simulink subsystem "F550_Dynamic_CA"  (R2024a)
settings: Solver=VariableStepAuto  StartTime=0.0  StopTime=10.0  RelTol=1e-3
values from neighbouring files (symbols this model uses):
  Jxx = 0.0211    [F550_data.m]
  Jyy = 0.0219    [F550_data.m]
  Jzz = 0.0366    [F550_data.m]
  Mass = 2.06    [F550_data.m]
settings Model: Creator=UASG  LastModifiedBy=UASG

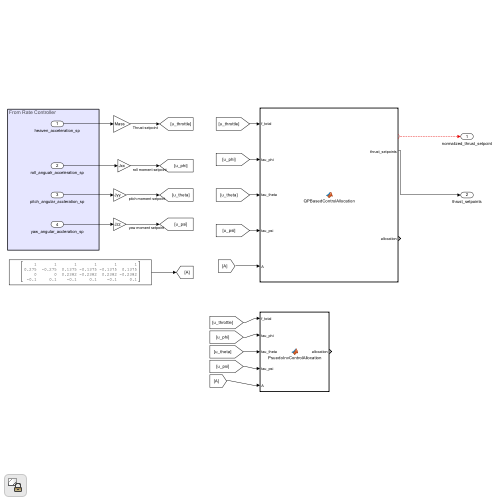
[thumbnail: Simulink's stored preview of the top-level diagram]
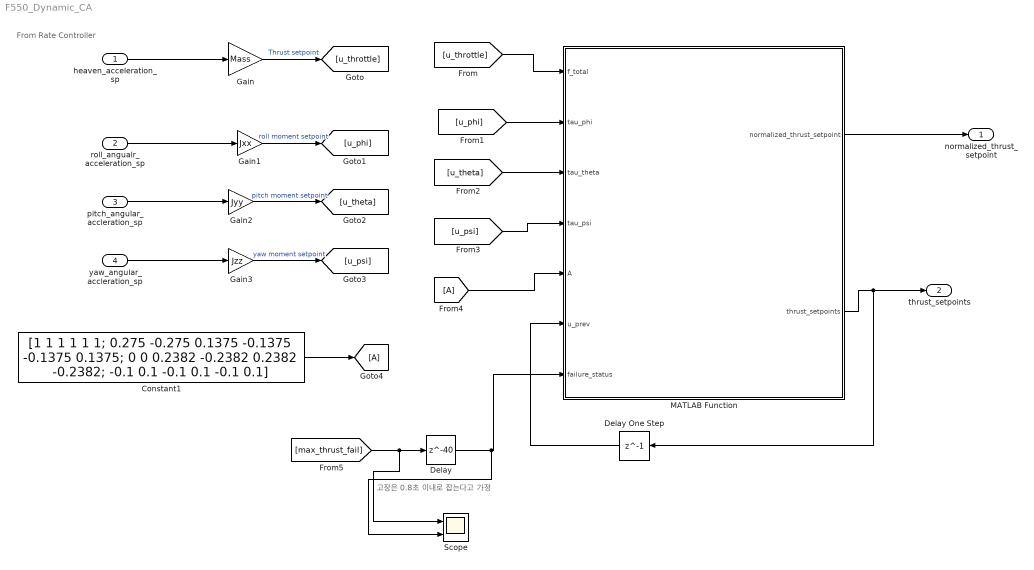
== system F550_Dynamic_CA ==
  note: 고장은 0.8초 이내로 잡는다고 가정
  note: From Rate Controller
  heaven_acceleration_sp : Inport
  roll_angualr_acceleration_sp : Inport  Port=2
  pitch_angular_accleration_sp : Inport  Port=3
  yaw_angular_accleration_sp : Inport  Port=4
  Constant1 : Constant  Value=[1 1 1 1 1 1; 0.275 -0.275 0.1375 -0.1375 -0.1375 0.1375; 0 0 0.2382 -0.2382 0.2382 -0.2382; -0.1 0.1 -0.1 0.1 -0.1 0.1]
  Delay : Delay  DelayLength=40  InitialCondition=1.0
  Delay One Step : Delay  DelayLength=1
  From4 : From
  Gain : Gain  Gain=Mass
  Gain1 : Gain  Gain=Jxx
  Gain2 : Gain  Gain=Jyy
  Gain3 : Gain  Gain=Jzz
  Goto4 : Goto
  MATLAB Function : MATLAB Function  TreatAsAtomicUnit=on
  Scope : Scope  NumInputPorts=2
  normalized_thrust_setpoint : Outport
  thrust_setpoints : Outport  Port=2
  wires:
  heaven_acceleration_sp/1 -> Gain/1
  roll_angualr_acceleration_sp/1 -> Gain1/1
  pitch_angular_accleration_sp/1 -> Gain2/1
  yaw_angular_accleration_sp/1 -> Gain3/1
  Constant1/1 -> Goto4/1
  MATLAB Function/1(normalized_thrust_setpoint) -> normalized_thrust_setpoint/1
  Gain/1 -> [u_throttle]  "Thrust setpoint"
  Gain1/1 -> [u_phi]  "roll moment setpoint"
  Gain2/1 -> [u_theta]  "pitch moment setpoint"
  Gain3/1 -> [u_psi]  "yaw moment setpoint"
  [u_phi] -> MATLAB Function/2(tau_phi)
  [u_throttle] -> MATLAB Function/1(f_total)
  [u_theta] -> MATLAB Function/3(tau_theta)
  [u_psi] -> MATLAB Function/4(tau_psi)
  From4/1 -> MATLAB Function/5(A)
  MATLAB Function/2(thrust_setpoints) -> thrust_setpoints/1, Delay One Step/1
  Delay One Step/1 -> MATLAB Function/6(u_prev)
  [max_thrust_fail] -> Delay/1, Scope/1
  Delay/1 -> MATLAB Function/7(failure_status), Scope/2

== matlab function F550_Dynamic_CA/MATLAB Function ==
  data: normalized_thrust_setpoint output; f_total input; thrust_setpoints output; tau_phi input; tau_theta input; tau_psi input; A input; u_prev input; failure_status input
function [normalized_thrust_setpoint, thrust_setpoints] = QPBasedControlAllocation(f_total, tau_phi, tau_theta, tau_psi, A, u_prev, failure_status)


% f_total: 추력 명령 [N], tau_phi, tau_theta, tau_psi: 롤 피치 요 토크 명령 [N.m]
% thrust_setpoints: 각 모터별 추력 명령[N] normalized_thrust_setpoint: 모터 최대 출력으로
% 정규화한 값
% A : Control Effectiviness MAtrix
num_actuator = 6;
u_des = [f_total; tau_phi; tau_theta; tau_psi];

% 각 추진기의 추력 제한 정의 (예시 값)
f_min = 0;           % 최소 추력 (뉴턴)
f_max = 5;           % 최대 추력 (뉴턴)

% 목적 함수의 이차 및 선형 계수 정의
% 목적: f' * f (추력의 제곱합 최소화)
H = 2 * eye(num_actuator);      % MATLAB의 quadprog은 (1/2)x'Hx + f'x를 최소화
f_obj = zeros(num_actuator,1);  % 선형 항 없음
%%
scenario = 2; 
numMotors = 6;
switch scenario
    case 1
        % 에너지 최소화: min u'u
        H = eye(numMotors);
        f_obj = zeros(numMotors,1); 
        
    case 2
        % 특정 모터 사용 억제: 모터 #1 가중치↑
        % H = diag([가중치,1,1,1,1,1])
        H = diag([1, 1, 1, 1, 1, 1]);
        f = zeros(numMotors,1);
        
    case 3
        % 추력 변화율 최소화: min (u - u_prev)'(u - u_prev)
        % = u'u - 2 u_prev'u + const
        % quadprog 형식: (1/2)*u'Hu + f'u -> 여기서 H = 2 * I, f = -2 * u_prev로 하면되지만
        % (1/2)을 빼려면 H=I로 하고 f=-2*u_prev을 그대로 써도 동일한 해를 얻기 위해,
        % 여기서는 H=I, f = -2*u_prev로 간단히 처리하겠습니다.
        
        % 실제 quadprog는 (1/2)*H*u'u + f'u를 최소화하므로
        % (1/2)*u'u + (-u_prev')*u = (1/2)*u'u - u_prev'*u
        % 이는 위 식과 상수항 차이만 있고 최소점 동일.
        H = eye(numMotors);
        f_obj = -2*u_prev; 
        % 정확히 하려면 H=2*eye(numMotors), f = -2*u_prev 로 두고,
        % 목적함수를 (1/2)*u'Hu + f'u 형태로 맞출 수 있음.
        % 여기서는 단순화해서 H=I, f=-2*u_prev 사용
        % 이 경우 목적함수는 (1/2)*u'u - u_prev'*u,
        % u'=u-u_prev일 때 상수항 무시하면 동일한 최소점.

        % 좀 더 엄밀히 하려면 다음과 같이 할 수도 있음:
        % H = 2*eye(numMotors);
        % f = -2*u_prev;
        % 이렇게 하면 목적함수는 (1/2)*u'(2I)u + (-2u_prev')u = u'u - u_prev'*u
        % = (u - u_prev)'(u - u_prev) - u_prev'u_prev (상수항 무시)
        % 이 경우가 더 직관적이므로 이렇게 하겠습니다.
        H = 2*eye(numMotors);
        f_obj = -2*u_prev;
end
%% QP
% 등식 제약 조건: A * f = u_des
Aeq = A;
beq = u_des;

failure_status = reshape(failure_status, 6, 1);

% 변수의 하한 및 상한
lb = f_min * [1 1 1 1 1 1]';
ub = f_max * failure_status;

% 이차 프로그래밍 문제 해결
options = optimoptions('quadprog', 'Display','none', 'Algorithm', 'active-set');  % 출력 숨기기
[thrust_setpoints, ~, ~, ~] = quadprog(H, f_obj, [], [], Aeq, beq, lb, ub, [0 0 0 0 0 0], options);
normalized_thrust_setpoint = thrust_setpoints ./ f_max;
